simulink model "Task3_state_observer_controller"  (R2023b)
settings: Solver=VariableStepAuto  StartTime=0.0  StopTime=1  RelTol=1e-3
values from neighbouring files (symbols this model uses):
  A = [-1.7  -0.25  0; 23  -30  20; 0  -250  -720]    [A.mat]
  B = [3  0; -103  0; 0  -790]    [B.mat]
  C = [0  1  0; 0  0  1]    [C.mat]
  K = K_bar*T    [Task1_pole_placement.m]    (also in Task2_LQR.m = R\B'*P; Task3_LQR_observer.m = R\B'*P; Task4_decoupling.m = F*[C(1,:)*(A+y11*eye(3));C(2,:)*(A+y21*eye(3))]; Task5_servo_control.m = R_ba\B_ba'*P)
  L = L_bar*T    [Task3_LQR_observer.m]    (also in Task5_servo_control.m)
settings Model: Creator=25039  LastModifiedBy=25039

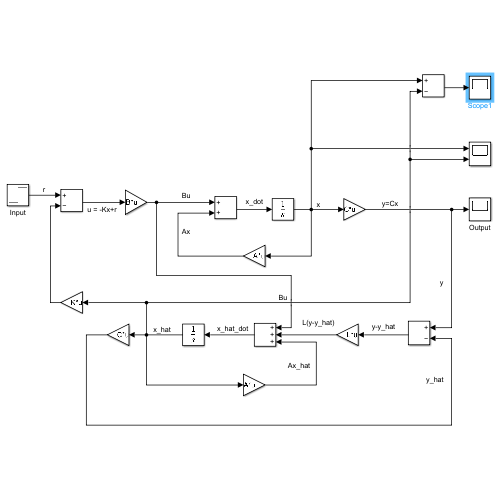
[thumbnail: Simulink's stored preview of the top-level diagram]
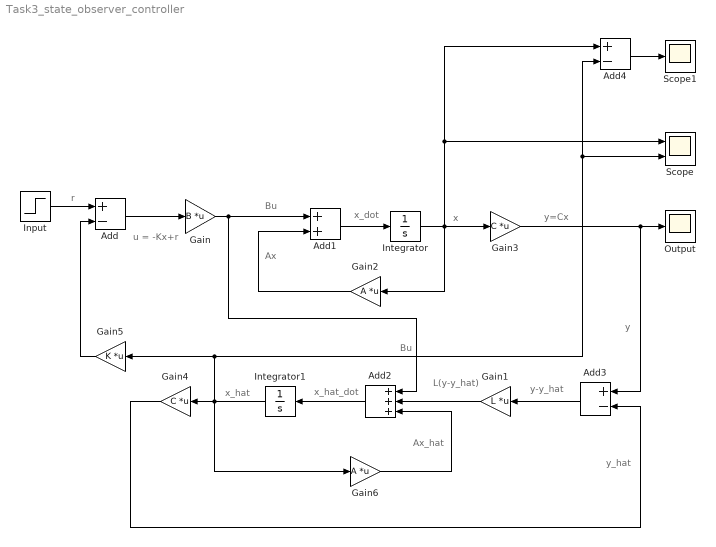
== system Task3_state_observer_controller ==
  note: y-y_hat
  note: L(y-y_hat)
  note: x_hat
  note: x_hat_dot
  note: y_hat
  note: y
  note: y=Cx
  note: x
  note: x_dot
  note: Ax
  note: Bu
  note: u = -Kx+r
  note: r
  note: Bu
  note: Ax_hat
  Add : Sum  Inputs=+-
  Add1 : Sum
  Add2 : Sum  Inputs=+++
  Add3 : Sum  Inputs=+-
  Add4 : Sum  Inputs=+-
  Gain : Gain  Gain=B  Multiplication=Matrix(K*u)
  Gain1 : Gain  Gain=L  Multiplication=Matrix(K*u)
  Gain2 : Gain  Gain=A  Multiplication=Matrix(K*u)
  Gain3 : Gain  Gain=C  Multiplication=Matrix(K*u)
  Gain4 : Gain  Gain=C  Multiplication=Matrix(K*u)
  Gain5 : Gain  Gain=K  Multiplication=Matrix(K*u)
  Gain6 : Gain  Gain=A  Multiplication=Matrix(K*u)
  Input : Step  Time=0  Before=[0, 0]  After=[0, 0]
  Integrator : Integrator  InitialCondition=[1,100,200]
  Integrator1 : Integrator
  Output : Scope
  Scope : Scope  NumInputPorts=2
  Scope1 : Scope
  wires:
  Input/1 -> Add/1
  Add/1 -> Gain/1
  Gain/1 -> Add2/1, Add1/1
  Add1/1 -> Integrator/1
  Gain3/1 -> Add3/1, Output/1
  Integrator/1 -> Add4/1, Scope/1, Gain2/1, Gain3/1
  Gain2/1 -> Add1/2
  Add3/1 -> Gain1/1
  Gain1/1 -> Add2/2
  Add2/1 -> Integrator1/1
  Integrator1/1 -> Gain6/1, Add4/2, Scope/2, Gain5/1, Gain4/1
  Gain5/1 -> Add/2
  Gain4/1 -> Add3/2
  Gain6/1 -> Add2/3
  Add4/1 -> Scope1/1
